simulink model "questao8"  (R2017a)
settings: Solver=VariableStepAuto  StartTime=0.0  StopTime=90  RelTol=1e-3
libraries: simulink x5
settings Model: Creator=julia  LastModifiedBy=julia

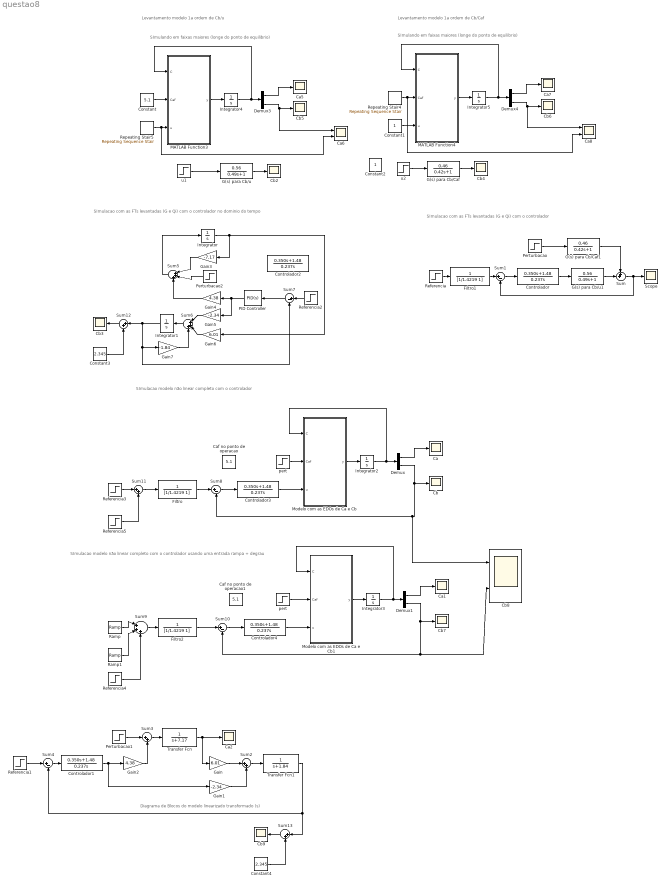
== system questao8 ==
  note: SImulacao modelo não linear completo com o controlador
  note: SImulando em faixas maiores (longe do ponto de equilibrio)
  note: Levantamento modelo 1a ordem de Cb/u
  note: Levantamento modelo 1a ordem de Cb/Caf
  note: SImulando em faixas maiores (longe do ponto de equilibrio)
  note: Diagrama de Blocos do modelo linearizado transformado (s)
  note: SImulacao com as FTs levantadas (G e Qi) com o controlador
  note: SImulacao com as FTs levantadas (G e Qi) com o controlador no dominio do tempo
  note: SImulacao modelo não linear completo com o controlador
      | usando uma entrada rampa + degrau
  Ca{,1..2,5,7} (5 alike) : Scope
  Ca6 : Scope  NumInputPorts=2
  Ca8 : Scope  NumInputPorts=2
  Caf no ponto de operacao : Constant  Value=5.1
  Caf no ponto de operacao1 : Constant  Value=5.1
  Cb{,2..7,9} (8 alike) : Scope
  Cb8 : Scope  NumInputPorts=2
  Constant : Constant  Value=5.1
  Constant1 : Constant
  Constant2 : Constant
  Constant3 : Constant  Value=2.345
  Constant4 : Constant  Value=2.345
  Controlador{,1..4} (5 alike) : TransferFcn  Numerator=[0.350 1.48]  Denominator=[0.237 0]
  Demux{,1,3..4} (4 alike) : Demux  Outputs=2
  Filtro : TransferFcn  Numerator=[0 1]  Denominator=[1/1.4219 1]
  Filtro1 : TransferFcn  Numerator=[0 1]  Denominator=[1/1.4219 1]
  Filtro2 : TransferFcn  Numerator=[0 1]  Denominator=[1/1.4219 1]
  G(s) para Cb/Caf : TransferFcn  Numerator=[0 0.46]  Denominator=[0.42 1]
  G(s) para Cb/Caf1 : TransferFcn  Numerator=[0 0.46]  Denominator=[0.42 1]
  G(s) para Cb/u : TransferFcn  Numerator=[0 0.56]  Denominator=[0.49 1]
  G(s) para Cb/u1 : TransferFcn  Numerator=[0 0.56]  Denominator=[0.49 1]
  Gain : Gain  Gain=6.01
  Gain1 : Gain  Gain=-2.34
  Gain2 : Gain  Gain=4.38
  Gain3 : Gain  Gain=-7.17
  Gain4 : Gain  Gain=4.38
  Gain5 : Gain  Gain=-2.34
  Gain6 : Gain  Gain=6.01
  Gain7 : Gain  Gain=-1.84
  Integrator : Integrator
  Integrator1 : Integrator
  Integrator{2..5} (4 alike) : Integrator  InitialCondition=[0.00001;0.00001]
  MATLAB Function3 : MATLAB Function  TreatAsAtomicUnit=on
  MATLAB Function4 : MATLAB Function  TreatAsAtomicUnit=on
  Modelo com as EDOs de Ca e Cb : MATLAB Function  TreatAsAtomicUnit=on
  Modelo com as EDOs de Ca e Cb1 : MATLAB Function  TreatAsAtomicUnit=on
  PID Controller : simulink/Continuous/PID Controller  Controller=PID  TimeDomain=Continuous-time  SampleTime=-1  IntegratorMethod=Forward Euler  FilterMethod=Forward Euler  Form=Parallel  UseFilter=on  ControllerParametersSource=internal  P=1.48  I=1.48/0.237  D=0  N=100  InitialConditionSource=internal  InitialConditionForIntegrator=0  InitialConditionForFilter=0  ExternalReset=none  LimitOutput=off  UpperSaturationLimit=inf  LowerSaturationLimit=-inf  LinearizeAsGain=on  AntiWindupMode=none  Kb=1  TrackingMode=off  Kt=1  PParamMin=[]  PParamMax=[]  IParamMin=[]  IParamMax=[]  DParamMin=[]  DParamMax=[]  NParamMin=[]  NParamMax=[]  KbParamMin=[]  KbParamMax=[]  KtParamMin=[]  KtParamMax=[]  POutMin=[]  POutMax=[]  IOutMin=[]  IOutMax=[]  DOutMin=[]  DOutMax=[]  NOutMin=[]  NOutMax=[]  KbOutMin=[]  KbOutMax=[]  KtOutMin=[]  KtOutMax=[]  IntegratorOutMin=[]  IntegratorOutMax=[]  FilterOutMin=[]  FilterOutMax=[]  SumOutMin=[]  SumOutMax=[]  SumI1OutMin=[]  SumI1OutMax=[]  SumI2OutMin=[]  SumI2OutMax=[]  SumI3OutMin=[]  SumI3OutMax=[]  SumDOutMin=[]  SumDOutMax=[]  SaturationOutMin=[]  SaturationOutMax=[]  IntegratorContinuousStateAttributes=''  IntegratorStateMustResolveToSignalObject=off  IntegratorRTWStateStorageClass=Auto  FilterContinuousStateAttributes=''  FilterStateMustResolveToSignalObject=off  FilterRTWStateStorageClass=Auto  DifferentiatorICPrevScaledInput=0  DifferentiatorOutMin=[]  DifferentiatorOutMax=[]  InitialConditionSetting=State (most efficient)
  Perturbacao : Step  Time=20  Before=4.5  After=4.6
  Perturbacao1 : Step  Time=80  After=0.2
  Perturbacao2 : Step  Time=0  After=0
  Ramp : simulink/Sources/Ramp  slope=2.345  start=0  X0=0
  Ramp1 : simulink/Sources/Ramp  slope=-2.345  start=1  X0=0
  Referencia : Step  Time=0  After=2.3
  Referencia1 : Step  Time=60  After=0.2
  Referencia2 : Step  Time=40  After=0.1
  Referencia3 : Step  Time=0  After=2.345
  Referencia4 : Step  Time=20  After=0.31
  Referencia5 : Step  Time=20  After=0.31
  Repeating Stair4 : simulink/Sources/Repeating Sequence Stair  OutValues=[4 4.15 4.3 4.45 4.6 4.75 4.9 5.05 5.2]  tsamp=10  OutMin=[]  OutMax=[]  OutDataTypeStr=double  OutputDataTypeScalingMode=double  OutDataType=fixdt(0,8)  ConRadixGroup=Best Precision: Vector-wise  OutScaling=2^-12
  Repeating Stair5 : simulink/Sources/Repeating Sequence Stair  OutValues=[0 0.15 0.30 0.45 0.6 0.75 0.9 1.05 1.2 1.35]  tsamp=10  OutMin=[]  OutMax=[]  OutDataTypeStr=double  OutputDataTypeScalingMode=double  OutDataType=fixdt(0,8)  ConRadixGroup=Best Precision: Vector-wise  OutScaling=2^-12
  Scope : Scope
  Sum : Sum  Inputs=++|
  Sum{1,4,7..8,10} (5 alike) : Sum  Inputs=|+-
  Sum{2..3,11..13} (5 alike) : Sum  Inputs=|++
  Sum5 : Sum  Inputs=|+++
  Sum6 : Sum  Inputs=|+++
  Sum9 : Sum  Inputs=|+++
  Transfer Fcn : TransferFcn  Denominator=[1 7.17]
  Transfer Fcn1 : TransferFcn  Denominator=[1 1.84]
  pert : Step  Time=40  Before=5.1  After=5.2
  "pert    " : Step  Time=60  Before=5.1  After=5.2
  u1 : Step  Time=0  After=1.1
  u2 : Step  Time=0  Before=4.5  After=5
  wires:
  Integrator2/1 -> Demux/1, Modelo com as EDOs de Ca e Cb/1(C)
  Modelo com as EDOs de Ca e Cb/1(y) -> Integrator2/1
  Demux/2 -> Cb/1, Cb8/1, Sum8/2
  Demux/1 -> Ca/1
  Controlador3/1 -> Modelo com as EDOs de Ca e Cb/3(u)
  u1/1 -> G(s) para Cb/u/1
  G(s) para Cb/u/1 -> Cb2/1
  G(s) para Cb/Caf/1 -> Cb4/1
  u2/1 -> G(s) para Cb/Caf/1
  Integrator4/1 -> Demux3/1, MATLAB Function3/1(C)
  MATLAB Function3/1(y) -> Integrator4/1
  Demux3/2 -> Cb5/1, Ca6/1
  Demux3/1 -> Ca5/1
  Repeating Stair5/1 -> MATLAB Function3/3(u), Ca6/2
  Constant/1 -> MATLAB Function3/2(Caf)
  Constant1/1 -> MATLAB Function4/3(u)
  Demux4/1 -> Ca7/1
  Demux4/2 -> Ca8/1, Cb6/1
  MATLAB Function4/1(y) -> Integrator5/1
  Integrator5/1 -> MATLAB Function4/1(C), Demux4/1
  Repeating Stair4/1 -> Ca8/2, MATLAB Function4/2(Caf)
  G(s) para Cb/Caf1/1 -> Sum/1
  G(s) para Cb/u1/1 -> Sum/2
  Controlador/1 -> G(s) para Cb/u1/1
  Perturbacao/1 -> G(s) para Cb/Caf1/1
  Sum/1 -> Sum1/2, Scope/1
  Sum1/1 -> Controlador/1
  Perturbacao1/1 -> Sum3/1
  Gain1/1 -> Sum2/2
  Gain2/1 -> Sum3/2
  Transfer Fcn/1 -> Ca2/1, Gain/1
  Sum2/1 -> Transfer Fcn1/1
  Sum3/1 -> Transfer Fcn/1
  Gain/1 -> Sum2/1
  Controlador1/1 -> Gain1/1, Gain2/1
  Sum4/1 -> Controlador1/1
  Referencia1/1 -> Sum4/1
  Integrator/1 -> Gain6/1, Gain3/1
  Gain3/1 -> Sum5/1
  Gain4/1 -> Sum5/3
  Gain5/1 -> Sum6/1
  Gain6/1 -> Sum6/2
  Sum5/1 -> Integrator/1
  Sum6/1 -> Integrator1/1
  Integrator1/1 -> Sum12/1, Sum7/2, Gain7/1
  Gain7/1 -> Sum6/3
  Referencia2/1 -> Sum7/1
  Perturbacao2/1 -> Sum5/2
  Sum8/1 -> Controlador3/1
  Filtro/1 -> Sum8/1
  Referencia/1 -> Filtro1/1
  Filtro1/1 -> Sum1/1
  Ramp/1 -> Sum9/1
  Ramp1/1 -> Sum9/2
  Sum10/1 -> Controlador4/1
  Controlador4/1 -> Modelo com as EDOs de Ca e Cb1/3(u)
  Demux1/1 -> Ca1/1
  Demux1/2 -> Cb8/2, Sum10/2, Cb7/1
  Modelo com as EDOs de Ca e Cb1/1(y) -> Integrator3/1
  Integrator3/1 -> Modelo com as EDOs de Ca e Cb1/1(C), Demux1/1
  Filtro2/1 -> Sum10/1
  Referencia4/1 -> Sum9/3
  Sum9/1 -> Filtro2/1
  Sum11/1 -> Filtro/1
  Referencia3/1 -> Sum11/1
  Referencia5/1 -> Sum11/2
  "pert    "/1 -> Modelo com as EDOs de Ca e Cb1/2(Caf)
  pert/1 -> Modelo com as EDOs de Ca e Cb/2(Caf)
  Sum12/1 -> Cb3/1
  Constant3/1 -> Sum12/2
  Transfer Fcn1/1 -> Sum13/1, Sum4/2
  Constant4/1 -> Sum13/2
  Sum13/1 -> Cb9/1
  PID Controller/1 -> Gain5/1, Gain4/1
  Sum7/1 -> PID Controller/1

== matlab function questao8/Modelo com as EDOs de Ca e Cb1 ==
  data: y output; C input; Caf input; u input
%EDOs das concentracoes dos produtos A e B
function y = fcn(C, Caf, u)

%constantes
k1 = 6.01; %L/min
k2 = 0.8433; %L/min
k3 = 0.1123; %mol/Lmin

%variaveis das concentracoes dos produtos A e B
Ca = C(1);
Cb = C(2);

%EDOs
Ca_d = -k1*Ca - k3*(Ca^2) + (Caf - Ca)*u;
Cb_d =  k1*Ca - k2*Cb - Cb*u;
 
%conjunto das EDOs
y = [Ca_d;Cb_d];

== matlab function questao8/Modelo com as EDOs de Ca e Cb ==
  data: y output; C input; Caf input; u input
%EDOs das concentracoes dos produtos A e B
function y = fcn(C, Caf, u)

%constantes
k1 = 6.01; %L/min
k2 = 0.8433; %L/min
k3 = 0.1123; %mol/Lmin

%variaveis das concentracoes dos produtos A e B
Ca = C(1);
Cb = C(2);

%EDOs
Ca_d = -k1*Ca - k3*(Ca^2) + (Caf - Ca)*u;
Cb_d =  k1*Ca - k2*Cb - Cb*u;
 
%conjunto das EDOs
y = [Ca_d;Cb_d];

== matlab function questao8/MATLAB Function3 ==
  data: y output; C input; Caf input; u input
%EDOs das concentracoes dos produtos A e B
function y = fcn(C, Caf, u)

%constantes
k1 = 6.01; %L/min
k2 = 0.8433; %L/min
k3 = 0.1123; %mol/Lmin

%variaveis das concentracoes dos produtos A e B
Ca = C(1);
Cb = C(2);

%EDOs
Ca_d = -k1*Ca - k3*(Ca^2) + (Caf - Ca)*u;
Cb_d =  k1*Ca - k2*Cb - Cb*u;
 
%conjunto das EDOs
y = [Ca_d;Cb_d];

== matlab function questao8/MATLAB Function4 ==
  data: y output; C input; Caf input; u input
%EDOs das concentracoes dos produtos A e B
function y = fcn(C, Caf, u)

%constantes
k1 = 6.01; %L/min
k2 = 0.8433; %L/min
k3 = 0.1123; %mol/Lmin

%variaveis das concentracoes dos produtos A e B
Ca = C(1);
Cb = C(2);

%EDOs
Ca_d = -k1*Ca - k3*(Ca^2) + (Caf - Ca)*u;
Cb_d =  k1*Ca - k2*Cb - Cb*u;
 
%conjunto das EDOs
y = [Ca_d;Cb_d];
